simulink library "ddm"  (R2021b)
settings: Solver=VariableStepAuto  StartTime=0.0  StopTime=10.0  RelTol=1e-3
undefined symbols (not defined in the file or in its folder): ADDM_FrTMTqDev_X_Nm, ADDM_RrTMTqDev_X_Nm, ENUM_ADASACCSTA_ERROR, ENUM_ADASACCSTA_OFF, ENUM_ADASACCSTA_STANDBY, ENUM_ALLOWMOV_ALLOWREADY, ENUM_APS, ENUM_BRKSTA_ERROR, ENUM_BRKSTA_OFF, ENUM_BRKSTA_ON, ENUM_BRKSW_INVALID, ENUM_BRKSW_OFF, ENUM_BRKSW_ON, ENUM_CHGPREACTERRSTA_OBCPRE, ENUM_DCDCFAULTSTA_ANYFAULTLV1, ENUM_DCDCFAULTSTA_ANYFAULTLV2, ENUM_DRIVETRAIN_AWD, ENUM_DRIVETRAIN_FWD, ENUM_DRIVETRAIN_RWD, ENUM_EDUDRTSTA_NORMAL, ENUM_EPBSTA_APPLIED, ENUM_EPBSTA_RELEASED, ENUM_ESCAPSSta_APSUNAVAILABLE, ENUM_GEARACTUALPOSN_INVALID, ENUM_GEARACTUALPOSN_P, ENUM_HVBATTREADYPRE_READY, ENUM_MCUWARN_LV0, ENUM_MCUWARN_LV1, ENUM_MCUWARN_LV2, ENUM_MCUWARN_LV3, ENUM_MCUWARN_NOERROR, ENUM_OBCFAULTSTA_ANYFAULT, ENUM_PAS_R2F2, ENUM_PDFAULT_BATTPDFAIL, ENUM_PDFAULT_DCDCDISABLE, ENUM_PDFAULT_MCUDISABLE, ENUM_PDFAULT_MCUDISCHRG, ENUM_POWERSTA_OFF, ENUM_POWERSTA_ON, ENUM_POWERSTA_READY, ENUM_POWERSTA_STANDBY, ENUM_PRESSINDI_LOW, ENUM_PUFAULT_BATTUPFAIL, ENUM_PUFAULT_DCDCENABLEFAIL, ENUM_PUFAULT_PRECHRGCHKFAIL, ENUM_PUFAULT_SAFETYCHKFAIL, ENUM_PUSTATE_COMPLETED, ENUM_PWRSTASW_OFF, ENUM_PWRSTASW_OFFA, ENUM_PWRSTASW_OFFCHVCHRG, ENUM_PWRSTASW_OFFCLVCHRG, ENUM_PWRSTASW_ON, ENUM_PWRSTASW_ONHVCHRG, ENUM_PWRSTASW_READY, ENUM_PWRSTASW_STANDBY, ENUM_RAPSErrWarnSta_NORMAL, ENUM_RAPSErrWarnSta_RAPSERRLV1, ENUM_SHIFTCOMMAND_P, ENUM_SHIFTERERRSTA_PBUTTONFAILURE, ENUM_VEHMALFUNLV_2ND ... (+463)
libraries: hcu_lib x529, $bdroot x5, simulink x4
(part 24 of 25)

== system ddm/DDM/DDM/VMC_DDM/FCM1/FCM1 Checksum Error  ==
  note: Test Detection Criteria
  note: Test Pass Criteria
  note: Release Condiction After Decision
  note: Diagnostics and Fault Handling
  task_time_s : Inport
  VDDM_FCM1CSErr_flg : Inport  Port=2
  No_CAN6_BUS_OFF : Inport  Port=3
  VDDM_FCM1NoComCFS_flg : Inport  Port=4
  VPMM_PowerSta_enum : Inport  Port=5
  DTC_clear_request : Inport  Port=6
  Constant : Constant  Value=ENUM_POWERSTA_OFF
  Constant1 : Constant  Value=FALSE
  Constant16 : Constant  Value=ZERO_INT
  Constant2 : Constant  Value=FALSE
  Constant3 : Constant  Value=KDDM_FCM1CSErrDTC_cnt
  Constant40 : Constant  Value=KDDM_FCM1CSErrDTC_cnt
  Constant41 : Constant  Value=KDDM_FCM1CSErrDetTO_s
  Constant49 : Constant  Value=ENUM_POWERSTA_OFF
  Constant5 : Constant  Value=ENUM_POWERSTA_OFF
  Constant52 : Constant  Value=ENUM_POWERSTA_STANDBY
  Constant6 : Constant  Value=KDDM_FCM1CSErrPassTO_s
  Constant7 : Constant  Value=TRUE
  Constant8 : Constant  Value=KDDM_VMCDiagnosisOffSW_flg
  Constant9 : Constant  Value=KDDM_FCM1CSErrPassTO_s
  DTC_Couter2 : hcu_lib/Basic_Blocks/DTC_Couter
  DTC_Info : hcu_lib/Basic_Blocks/DTC_Info
  Equal : RelationalOperator  Operator=~=  OutDataTypeStr=boolean  RndMeth=Simplest
  Equal1 : RelationalOperator  Operator===  OutDataTypeStr=boolean  RndMeth=Simplest
  Equal2 : RelationalOperator  Operator=~=  OutDataTypeStr=boolean  RndMeth=Simplest
  Equal3 : RelationalOperator  OutDataTypeStr=boolean  RndMeth=Simplest
  Equal8 : RelationalOperator  Operator===  OutDataTypeStr=boolean  RndMeth=Simplest
  Logical Operator1 : Logic  Operator=NOT  AllPortsSameDT=off  OutDataTypeStr=boolean
  Logical Operator10 : Logic  Operator=OR  Inputs=4  AllPortsSameDT=off  OutDataTypeStr=boolean
  Logical Operator11 : Logic  AllPortsSameDT=off  OutDataTypeStr=boolean
  Logical Operator16 : Logic  Operator=NOT  AllPortsSameDT=off  OutDataTypeStr=boolean
  Logical Operator2 : Logic  Inputs=3  AllPortsSameDT=off  OutDataTypeStr=boolean
  Logical Operator4 : Logic  Inputs=3  AllPortsSameDT=off  OutDataTypeStr=boolean
  Logical Operator6 : Logic  Operator=NOT  AllPortsSameDT=off  OutDataTypeStr=boolean
  Relational Operator : RelationalOperator  Operator=>  OutDataTypeStr=boolean  RndMeth=Simplest
  Switch2 : Switch  Criteria=u2 ~= 0
  Switch3 : Switch  Criteria=u2 ~= 0
  Switch5 : Switch  Criteria=u2 ~= 0
  Terminator1 : Terminator
  Test Detection Criteria : hcu_lib/Basic_Blocks/Test Detection Criteria
  Timer1 : hcu_lib/Basic_Blocks/Timer
  Unit Delay3 : UnitDelay  SampleTime=-1  HasFrameUpgradeWarning=on
  VDDM_FCM1CSErrCFS_flg : Outport
  VDDM_FCM1CSErrDTC_raw32 : Outport  Port=2
  wires:
  Relational Operator/1 -> Terminator1/1  "VDDM_FCM1CSErrDFS_flg"
  DTC_Couter2/1 -> [VDDM_FCM1CSErrCFS_flg]  "VDDM_FCM1CSErrCFS_flg"
  [VPMM_PowerSta_enum] -> Unit Delay3/1
  Logical Operator10/1 -> [VDDM_FCM1CSErrCFSRls_flg]  "VDDM_FCM1CSErrCFSRls_flg"
  [VPMM_PowerSta_enum] -> Equal8/1
  [DTC_clear_request] -> Logical Operator10/2
  [VDDM_FCM1CSErrPass_flg] -> Logical Operator10/3
  Constant8/1 -> Logical Operator10/4
  Equal1/1 -> Logical Operator11/1
  Logical Operator11/1 -> Logical Operator10/1
  Unit Delay3/1 -> Equal1/1
  Constant52/1 -> Equal8/2
  DTC_Couter2/2 -> Relational Operator/1  "VDDM_FCM1CSErrDTC_cnt"
  Equal8/1 -> Logical Operator11/2
  Constant49/1 -> Equal1/2
  Constant16/1 -> Relational Operator/2
  Constant3/1 -> DTC_Couter2/3
  [VDDM_FCM1CSErrCFSRls_flg] -> DTC_Couter2/2
  [VDDM_FCM1CSErrDet_flg] -> DTC_Couter2/1
  DTC_Info/1 -> VDDM_FCM1CSErrDTC_raw32/1
  [DTC_clear_request] -> DTC_Info/4
  [VDDM_FCM1CSErrCFS_flg] -> DTC_Info/3
  [VDDM_FCM1CSErrPass_flg] -> DTC_Info/2
  [VDDM_FCM1CSErrDet_flg] -> DTC_Info/1
  Switch5/1 -> Test Detection Criteria/1
  [VDDM_FCM1CSErrCFSRls_flg] -> Switch5/2
  Constant1/1 -> Switch5/1
  Switch2/1 -> Switch5/3
  [task_time_s] -> Timer1/3
  VDDM_FCM1NoComCFS_flg/1 -> [VDDM_FCM1NoComCFS_flg]
  [No_CAN6_BUS_OFF] -> Logical Operator2/1
  Logical Operator16/1 -> Logical Operator2/2
  [VDDM_FCM1NoComCFS_flg] -> Logical Operator16/1
  Constant9/1 -> Timer1/4
  task_time_s/1 -> [task_time_s]  "task_time_s"
  Constant40/1 -> Test Detection Criteria/3
  Constant6/1 -> Equal3/2
  Equal3/1 -> [VDDM_FCM1CSErrPass_flg]  "VDDM_FCM1CSErrPass_flg"
  Equal/1 -> Logical Operator2/3
  Equal2/1 -> Logical Operator4/2
  [No_CAN6_BUS_OFF] -> Logical Operator4/1
  [VPMM_PowerSta_enum] -> Equal2/1
  [VDDM_FCM1CSErr_flg] -> Switch3/1
  Constant/1 -> Equal/2
  Switch3/1 -> Timer1/2, Logical Operator6/1
  [VPMM_PowerSta_enum] -> Equal/1
  Constant41/1 -> Test Detection Criteria/4
  [task_time_s] -> Test Detection Criteria/2
  Test Detection Criteria/1 -> [VDDM_FCM1CSErrDet_flg]  "VDDM_FCM1CSErrDet_flg"
  Logical Operator2/1 -> Switch2/2
  Timer1/1 -> Equal3/1
  [VDDM_FCM1CSErr_flg] -> Switch2/1
  Constant7/1 -> Switch3/3
  Logical Operator4/1 -> Switch3/2
  Constant2/1 -> Switch2/3
  Constant5/1 -> Equal2/2
  Logical Operator6/1 -> Timer1/1
  [VDDM_FCM1CSErrCFS_flg] -> VDDM_FCM1CSErrCFS_flg/1
  VDDM_FCM1CSErr_flg/1 -> [VDDM_FCM1CSErr_flg]
  No_CAN6_BUS_OFF/1 -> [No_CAN6_BUS_OFF]
  DTC_clear_request/1 -> [DTC_clear_request]
  VPMM_PowerSta_enum/1 -> [VPMM_PowerSta_enum]
  Logical Operator1/1 -> Logical Operator4/3
  [VDDM_FCM1NoComCFS_flg] -> Logical Operator1/1

== system ddm/DDM/DDM/VMC_DDM/FCM1/FCM1 Lost Com ==
  note: Release Condiction After Decision
  note: Diagnostics and Fault Handling
  note: Test Detection Criteria
  note: Test Pass Criteria
  task_time_s : Inport
  VDDM_FCM1NoCom_flg : Inport  Port=2
  No_CAN6_BUS_OFF : Inport  Port=3
  VPMM_PowerSta_enum : Inport  Port=4
  DTC_clear_request : Inport  Port=5
  Constant : Constant  Value=ENUM_POWERSTA_OFF
  Constant1 : Constant  Value=FALSE
  Constant10 : Constant  Value=KDDM_FCM1NoComDTC_cnt
  Constant2 : Constant  Value=FALSE
  Constant3 : Constant  Value=KDDM_VMCDiagnosisOffSW_flg
  Constant40 : Constant  Value=KDDM_FCM1NoComDTC_cnt
  Constant41 : Constant  Value=KDDM_FCM1NoComDetTO_s
  Constant49 : Constant  Value=ENUM_POWERSTA_OFF
  Constant5 : Constant  Value=ENUM_POWERSTA_OFF
  Constant52 : Constant  Value=ENUM_POWERSTA_STANDBY
  Constant6 : Constant  Value=KDDM_FCM1NoComPassTO_s
  Constant7 : Constant  Value=TRUE
  Constant8 : Constant  Value=ZERO_INT
  Constant9 : Constant  Value=KDDM_FCM1NoComPassTO_s
  DTC_Couter2 : hcu_lib/Basic_Blocks/DTC_Couter
  DTC_Info : hcu_lib/Basic_Blocks/DTC_Info
  Equal : RelationalOperator  Operator=~=  OutDataTypeStr=boolean  RndMeth=Simplest
  Equal1 : RelationalOperator  Operator===  OutDataTypeStr=boolean  RndMeth=Simplest
  Equal2 : RelationalOperator  Operator=~=  OutDataTypeStr=boolean  RndMeth=Simplest
  Equal3 : RelationalOperator  OutDataTypeStr=boolean  RndMeth=Simplest
  Equal8 : RelationalOperator  Operator===  OutDataTypeStr=boolean  RndMeth=Simplest
  Logical Operator10 : Logic  Operator=OR  Inputs=4  AllPortsSameDT=off  OutDataTypeStr=boolean
  Logical Operator11 : Logic  AllPortsSameDT=off  OutDataTypeStr=boolean
  Logical Operator2 : Logic  AllPortsSameDT=off  OutDataTypeStr=boolean
  Logical Operator4 : Logic  AllPortsSameDT=off  OutDataTypeStr=boolean
  Logical Operator6 : Logic  Operator=NOT  AllPortsSameDT=off  OutDataTypeStr=boolean
  Relational Operator : RelationalOperator  Operator=>  OutDataTypeStr=boolean  RndMeth=Simplest
  Switch2 : Switch  Criteria=u2 ~= 0
  Switch3 : Switch  Criteria=u2 ~= 0
  Switch5 : Switch  Criteria=u2 ~= 0
  Terminator : Terminator
  Test Detection Criteria : hcu_lib/Basic_Blocks/Test Detection Criteria
  Timer1 : hcu_lib/Basic_Blocks/Timer
  Unit Delay3 : UnitDelay  SampleTime=-1  HasFrameUpgradeWarning=on
  VDDM_FCM1NoComCFS_flg : Outport
  VDDM_FCM1NoComDTC_raw32 : Outport  Port=2
  wires:
  [VDDM_FCM1NoComPass_flg] -> Logical Operator10/3
  Constant10/1 -> DTC_Couter2/3
  [VDDM_FCM1NoComCFSRls_flg] -> DTC_Couter2/2
  [VDDM_FCM1NoComDet_flg] -> DTC_Couter2/1
  Relational Operator/1 -> Terminator/1  "VDDM_FCM1NoComDFS_flg"
  DTC_Couter2/1 -> [VDDM_FCM1NoComCFS_flg]  "VDDM_FCM1NoComCFS_flg"
  [VPMM_PowerSta_enum] -> Equal8/1
  [DTC_clear_request] -> Logical Operator10/2
  Equal8/1 -> Logical Operator11/2
  [VPMM_PowerSta_enum] -> Unit Delay3/1
  Logical Operator10/1 -> [VDDM_FCM1NoComCFSRls_flg]  "VDDM_FCM1NoComCFSRls_flg"
  Logical Operator11/1 -> Logical Operator10/1
  Constant49/1 -> Equal1/2
  Unit Delay3/1 -> Equal1/1
  Equal1/1 -> Logical Operator11/1
  DTC_Couter2/2 -> Relational Operator/1  "VDDM_FCM1NoComDTC_cnt"
  Constant3/1 -> Logical Operator10/4
  Constant52/1 -> Equal8/2
  Constant8/1 -> Relational Operator/2
  DTC_Info/1 -> VDDM_FCM1NoComDTC_raw32/1
  [DTC_clear_request] -> DTC_Info/4
  [VDDM_FCM1NoComCFS_flg] -> DTC_Info/3
  [VDDM_FCM1NoComPass_flg] -> DTC_Info/2
  [VDDM_FCM1NoComDet_flg] -> DTC_Info/1
  Constant1/1 -> Switch5/1
  [VDDM_FCM1NoComCFSRls_flg] -> Switch5/2
  Switch5/1 -> Test Detection Criteria/1
  [task_time_s] -> Timer1/3
  Constant9/1 -> Timer1/4
  task_time_s/1 -> [task_time_s]  "task_time_s"
  Constant40/1 -> Test Detection Criteria/3
  Constant6/1 -> Equal3/2
  Equal3/1 -> [VDDM_FCM1NoComPass_flg]  "VDDM_FCM1NoComPass_flg"
  Equal/1 -> Logical Operator2/2
  Equal2/1 -> Logical Operator4/2
  [No_CAN6_BUS_OFF] -> Logical Operator4/1
  [VPMM_PowerSta_enum] -> Equal2/1
  [VDDM_FCM1NoCom_flg] -> Switch3/1
  Switch2/1 -> Switch5/3
  Constant/1 -> Equal/2
  Switch3/1 -> Timer1/2, Logical Operator6/1
  [VPMM_PowerSta_enum] -> Equal/1
  Constant41/1 -> Test Detection Criteria/4
  [task_time_s] -> Test Detection Criteria/2
  Test Detection Criteria/1 -> [VDDM_FCM1NoComDet_flg]  "VDDM_FCM1NoComDet_flg"
  Logical Operator2/1 -> Switch2/2
  Timer1/1 -> Equal3/1
  [VDDM_FCM1NoCom_flg] -> Switch2/1
  Constant7/1 -> Switch3/3
  Logical Operator4/1 -> Switch3/2
  Constant2/1 -> Switch2/3
  Constant5/1 -> Equal2/2
  [No_CAN6_BUS_OFF] -> Logical Operator2/1
  Logical Operator6/1 -> Timer1/1
  [VDDM_FCM1NoComCFS_flg] -> VDDM_FCM1NoComCFS_flg/1
  VDDM_FCM1NoCom_flg/1 -> [VDDM_FCM1NoCom_flg]
  No_CAN6_BUS_OFF/1 -> [No_CAN6_BUS_OFF]
  DTC_clear_request/1 -> [DTC_clear_request]
  VPMM_PowerSta_enum/1 -> [VPMM_PowerSta_enum]

== system ddm/DDM/DDM/VMC_DDM/FCM1/FCM1 Rolling Count Error  ==
  note: Test Detection Criteria
  note: Test Pass Criteria
  note: Release Condiction After Decision
  note: Diagnostics and Fault Handling
  task_time_s : Inport
  VDDM_FCM1RCErr_flg : Inport  Port=2
  No_CAN6_BUS_OFF : Inport  Port=3
  VDDM_FCM1NoComCFS_flg : Inport  Port=4
  VPMM_PowerSta_enum : Inport  Port=5
  DTC_clear_request : Inport  Port=6
  Constant : Constant  Value=ENUM_POWERSTA_OFF
  Constant1 : Constant  Value=FALSE
  Constant16 : Constant  Value=ZERO_INT
  Constant2 : Constant  Value=FALSE
  Constant3 : Constant  Value=KDDM_FCM1RCErrDTC_cnt
  Constant40 : Constant  Value=KDDM_FCM1RCErrDTC_cnt
  Constant41 : Constant  Value=KDDM_FCM1RCErrDetTO_s
  Constant49 : Constant  Value=ENUM_POWERSTA_OFF
  Constant5 : Constant  Value=ENUM_POWERSTA_OFF
  Constant52 : Constant  Value=ENUM_POWERSTA_STANDBY
  Constant6 : Constant  Value=KDDM_FCM1RCErrPassTO_s
  Constant7 : Constant  Value=TRUE
  Constant8 : Constant  Value=KDDM_VMCDiagnosisOffSW_flg
  Constant9 : Constant  Value=KDDM_FCM1RCErrPassTO_s
  DTC_Couter2 : hcu_lib/Basic_Blocks/DTC_Couter
  DTC_Info : hcu_lib/Basic_Blocks/DTC_Info
  Equal : RelationalOperator  Operator=~=  OutDataTypeStr=boolean  RndMeth=Simplest
  Equal1 : RelationalOperator  Operator===  OutDataTypeStr=boolean  RndMeth=Simplest
  Equal2 : RelationalOperator  Operator=~=  OutDataTypeStr=boolean  RndMeth=Simplest
  Equal3 : RelationalOperator  OutDataTypeStr=boolean  RndMeth=Simplest
  Equal8 : RelationalOperator  Operator===  OutDataTypeStr=boolean  RndMeth=Simplest
  From6 : From  Commented=on  GotoTag=VDDM_EDriveSysErrVCUErr_flg
  Logical Operator10 : Logic  Operator=OR  Inputs=4  AllPortsSameDT=off  OutDataTypeStr=boolean
  Logical Operator11 : Logic  AllPortsSameDT=off  OutDataTypeStr=boolean
  Logical Operator16 : Logic  Operator=NOT  AllPortsSameDT=off  OutDataTypeStr=boolean
  Logical Operator2 : Logic  Inputs=3  AllPortsSameDT=off  OutDataTypeStr=boolean
  Logical Operator4 : Logic  AllPortsSameDT=off  OutDataTypeStr=boolean
  Logical Operator6 : Logic  Operator=NOT  AllPortsSameDT=off  OutDataTypeStr=boolean
  Relational Operator : RelationalOperator  Operator=>  OutDataTypeStr=boolean  RndMeth=Simplest
  Switch2 : Switch  Criteria=u2 ~= 0
  Switch3 : Switch  Criteria=u2 ~= 0
  Switch5 : Switch  Criteria=u2 ~= 0
  Terminator : Terminator
  Terminator1 : Terminator
  Test Detection Criteria : hcu_lib/Basic_Blocks/Test Detection Criteria
  Timer1 : hcu_lib/Basic_Blocks/Timer
  Unit Delay3 : UnitDelay  SampleTime=-1  HasFrameUpgradeWarning=on
  VDDM_FCM1RCErrCFS_flg : Outport
  VDDM_FCM1RCErrDTC_raw32 : Outport  Port=2
  wires:
  Relational Operator/1 -> Terminator1/1  "VDDM_FCM1RCErrDFS_flg"
  Constant3/1 -> DTC_Couter2/3
  Equal8/1 -> Logical Operator11/2
  Constant16/1 -> Relational Operator/2
  [VDDM_FCM1RCErrPass_flg] -> Logical Operator10/3
  [VDDM_FCM1RCErrCFSRls_flg] -> DTC_Couter2/2
  Logical Operator10/1 -> [VDDM_FCM1RCErrCFSRls_flg]  "VDDM_FCM1RCErrCFSRls_flg"
  [VDDM_FCM1RCErrDet_flg] -> DTC_Couter2/1
  Constant52/1 -> Equal8/2
  DTC_Couter2/2 -> Relational Operator/1  "VDDM_FCM1RCErrDTC_cnt"
  Constant49/1 -> Equal1/2
  Logical Operator11/1 -> Logical Operator10/1
  Unit Delay3/1 -> Equal1/1
  Equal1/1 -> Logical Operator11/1
  Constant8/1 -> Logical Operator10/4
  [VPMM_PowerSta_enum] -> Equal8/1
  [DTC_clear_request] -> Logical Operator10/2
  [VPMM_PowerSta_enum] -> Unit Delay3/1
  DTC_Couter2/1 -> [VDDM_FCM1RCErrCFS_flg]  "VDDM_FCM1RCErrCFS_flg"
  DTC_Info/1 -> VDDM_FCM1RCErrDTC_raw32/1
  [DTC_clear_request] -> DTC_Info/4
  [VDDM_FCM1RCErrCFS_flg] -> DTC_Info/3
  [VDDM_FCM1RCErrPass_flg] -> DTC_Info/2
  [VDDM_FCM1RCErrDet_flg] -> DTC_Info/1
  Switch5/1 -> Test Detection Criteria/1
  Constant1/1 -> Switch5/1
  [VDDM_FCM1RCErrCFSRls_flg] -> Switch5/2
  [task_time_s] -> Timer1/3
  VDDM_FCM1NoComCFS_flg/1 -> [VDDM_FCM1NoComCFS_flg]
  [No_CAN6_BUS_OFF] -> Logical Operator2/1
  Logical Operator16/1 -> Logical Operator2/2
  [VDDM_FCM1NoComCFS_flg] -> Logical Operator16/1
  Constant9/1 -> Timer1/4
  task_time_s/1 -> [task_time_s]  "task_time_s"
  Constant40/1 -> Test Detection Criteria/3
  Constant6/1 -> Equal3/2
  Equal3/1 -> [VDDM_FCM1RCErrPass_flg]  "VDDM_FCM1RCErrPass_flg"
  Equal/1 -> Logical Operator2/3
  Equal2/1 -> Logical Operator4/2
  [No_CAN6_BUS_OFF] -> Logical Operator4/1
  [VPMM_PowerSta_enum] -> Equal2/1
  [VDDM_FCM1RCErr_flg] -> Switch3/1
  Switch2/1 -> Switch5/3
  Constant/1 -> Equal/2
  Switch3/1 -> Timer1/2, Logical Operator6/1
  [VPMM_PowerSta_enum] -> Equal/1
  Constant41/1 -> Test Detection Criteria/4
  [task_time_s] -> Test Detection Criteria/2
  Test Detection Criteria/1 -> [VDDM_FCM1RCErrDet_flg]  "VDDM_FCM1RCErrDet_flg"
  Logical Operator2/1 -> Switch2/2
  Timer1/1 -> Equal3/1
  [VDDM_FCM1RCErr_flg] -> Switch2/1
  Constant7/1 -> Switch3/3
  Logical Operator4/1 -> Switch3/2
  Constant2/1 -> Switch2/3
  Constant5/1 -> Equal2/2
  Logical Operator6/1 -> Timer1/1
  From6/1 -> Terminator/1
  [VDDM_FCM1RCErrCFS_flg] -> VDDM_FCM1RCErrCFS_flg/1
  VDDM_FCM1RCErr_flg/1 -> [VDDM_FCM1RCErr_flg]
  No_CAN6_BUS_OFF/1 -> [No_CAN6_BUS_OFF]
  DTC_clear_request/1 -> [DTC_clear_request]
  VPMM_PowerSta_enum/1 -> [VPMM_PowerSta_enum]

== system ddm/DDM/DDM/VMC_DDM/FCMACC Signal Error/FCMACC Signal Error  ==
  note: Test Detection Criteria
  note: Test Pass Criteria
  note: Diagnostics and Fault Handling
  note: Release Condiction After Decision
  task_time_s : Inport
  VDDM_FCM1NoComCFS_flg : Inport  Port=2
  VDDM_FCM1RCErrCFS_flg : Inport  Port=3
  VDDM_FCM1CSErrCFS_flg : Inport  Port=4
  No_CAN6_BUS_OFF : Inport  Port=5
  VPMM_PowerSta_enum : Inport  Port=6
  VINP_ADASACCSta_enum : Inport  Port=7
  DTC_clear_request : Inport  Port=8
  VTQD_ExternalTqAllow_flg : Inport  Port=9
  VTQD_ExtDoorAllow_flg : Inport  Port=10
  AND : Logic  Inputs=3  AllPortsSameDT=off  OutDataTypeStr=boolean
  Constant : Constant  Value=ENUM_POWERSTA_OFF
  Constant1 : Constant  Value=ENUM_POWERSTA_OFF
  Constant10 : Constant  Value=ZERO_INT
  Constant12 : Constant  Value=KDDM_FCMACCSigErrDTC_cnt
  Constant16 : Constant  Value=ENUM_ADASACCSTA_STANDBY
  Constant18 : Constant  Value=ENUM_POWERSTA_OFF
  Constant{2,5,19,24} (4 alike) : Constant  Value=FALSE
  Constant20 : Constant  Value=ENUM_POWERSTA_STANDBY
  Constant21 : Constant  Value=TRUE
  Constant25 : Constant  Value=KDDM_VMCDiagnosisOffSW_flg
  Constant3 : Constant  Value=ENUM_ADASACCSTA_ERROR
  Constant4 : Constant  Value=KDDM_FCMACCSigErrDetTO_s
  Constant6 : Constant  Value=KDDM_FCMACCSigErrPassTO_s
  Constant7 : Constant  Value=KDDM_FCMACCSigErrDTC_cnt
  Constant8 : Constant  Value=ENUM_ADASACCSTA_OFF
  Constant9 : Constant  Value=KDDM_FCMACCSigErrPassTO_s
  DTC_Couter1 : hcu_lib/Basic_Blocks/DTC_Couter
  DTC_Info : hcu_lib/Basic_Blocks/DTC_Info
  Equal : RelationalOperator  Operator=~=  OutDataTypeStr=boolean  RndMeth=Simplest
  Equal1 : RelationalOperator  Operator=~=  OutDataTypeStr=boolean  RndMeth=Simplest
  Equal{2,4..5,8..9} (5 alike) : RelationalOperator  Operator===  OutDataTypeStr=boolean  RndMeth=Simplest
  Equal3 : RelationalOperator  OutDataTypeStr=boolean  RndMeth=Simplest
  Logical Operator1 : Logic  Operator=OR  Inputs=4  AllPortsSameDT=off  OutDataTypeStr=boolean
  Logical Operator10 : Logic  AllPortsSameDT=off  OutDataTypeStr=boolean
  Logical Operator{3,5,11..12,14,17..18} (7 alike) : Logic  Operator=NOT  AllPortsSameDT=off  OutDataTypeStr=boolean
  Logical Operator13 : Logic  Inputs=5  AllPortsSameDT=off  OutDataTypeStr=boolean
  Logical Operator2 : Logic  Inputs=5  AllPortsSameDT=off  OutDataTypeStr=boolean
  Logical Operator4 : Logic  Operator=OR  AllPortsSameDT=off  OutDataTypeStr=boolean
  Relational Operator : RelationalOperator  Operator=>  OutDataTypeStr=boolean  RndMeth=Simplest
  Switch{2..3,5..6} (4 alike) : Switch  Criteria=u2 ~= 0
  Terminator : Terminator
  Test Detection Criteria : hcu_lib/Basic_Blocks/Test Detection Criteria
  Timer1 : hcu_lib/Basic_Blocks/Timer
  Unit Delay1 : UnitDelay  SampleTime=-1  HasFrameUpgradeWarning=on
  VDDM_FCMACCSigErrCFS_flg : Outport
  VDDM_FCMACCSigErrDetDTC_raw32 : Outport  Port=2
  wires:
  Switch2/1 -> Switch5/3
  Equal3/1 -> [VDDM_FCMACCSigErrPass_flg]  "VDDM_FCMACCSigErrPass_flg"
  [VDDM_FCMACCSigErrCFS_flg] -> VDDM_FCMACCSigErrCFS_flg/1
  Constant6/1 -> Equal3/2
  [No_CAN6_BUS_OFF] -> Logical Operator2/1
  Logical Operator2/1 -> Switch2/2
  Switch3/1 -> Timer1/1, Logical Operator14/1
  Constant2/1 -> Switch2/3
  Timer1/1 -> Equal3/1
  VDDM_FCM1NoComCFS_flg/1 -> [VDDM_FCM1NoComCFS_flg]
  DTC_clear_request/1 -> [DTC_clear_request]
  VDDM_FCM1CSErrCFS_flg/1 -> [VDDM_FCM1CSErrCFS_flg]
  VPMM_PowerSta_enum/1 -> [VPMM_PowerSta_enum]
  No_CAN6_BUS_OFF/1 -> [No_CAN6_BUS_OFF]
  [VDDM_FCM1NoComCFS_flg] -> Logical Operator17/1
  [VDDM_FCM1CSErrCFS_flg] -> Logical Operator18/1
  Logical Operator17/1 -> Logical Operator2/2
  Logical Operator18/1 -> Logical Operator2/4
  Logical Operator13/1 -> Switch3/2
  Constant5/1 -> Switch3/3
  task_time_s/1 -> [task_time_s]  "task_time_s"
  [task_time_s] -> Test Detection Criteria/2
  Constant7/1 -> Test Detection Criteria/3
  Test Detection Criteria/1 -> [VDDM_FCMACCSigErrDet_flg]  "VDDM_FCMACCSigErrDet_flg"
  Constant9/1 -> Timer1/4
  Equal/1 -> Logical Operator2/5
  VINP_ADASACCSta_enum/1 -> [VINP_ADASACCSta_enum]
  [VINP_ADASACCSta_enum] -> Equal5/1
  Constant3/1 -> Equal5/2
  [VINP_ADASACCSta_enum] -> Equal8/1
  Equal8/1 -> Logical Operator4/1
  Constant8/1 -> Equal8/2
  Logical Operator4/1 -> Switch3/1
  Constant16/1 -> Equal9/2
  [VINP_ADASACCSta_enum] -> Equal9/1
  Equal9/1 -> Logical Operator4/2
  [VDDM_FCM1CSErrCFS_flg] -> Logical Operator12/1
  Logical Operator11/1 -> Logical Operator13/2
  [No_CAN6_BUS_OFF] -> Logical Operator13/1
  [VDDM_FCM1NoComCFS_flg] -> Logical Operator11/1
  Equal1/1 -> Logical Operator13/5
  Logical Operator12/1 -> Logical Operator13/4
  Logical Operator14/1 -> Timer1/2
  [VDDM_FCMACCSigErrCFSRls_flg] -> Switch5/2
  Constant19/1 -> Switch5/1
  Switch5/1 -> Test Detection Criteria/1
  [VDDM_FCMACCSigErrDet_flg] -> DTC_Info/1
  [VDDM_FCMACCSigErrPass_flg] -> DTC_Info/2
  [VDDM_FCMACCSigErrCFS_flg] -> DTC_Info/3
  [DTC_clear_request] -> DTC_Info/4
  DTC_Info/1 -> VDDM_FCMACCSigErrDetDTC_raw32/1  "VDDM_FCMACCSigErrDetDTC_raw32"
  VTQD_ExtDoorAllow_flg/1 -> [VTQD_ExtDoorAllow_flg]
  VTQD_ExternalTqAllow_flg/1 -> [VTQD_ExternalTqAllow_flg]
  AND/1 -> Switch2/1
  Equal5/1 -> AND/2
  [VTQD_ExtDoorAllow_flg] -> AND/3
  [VTQD_ExternalTqAllow_flg] -> AND/1
  Constant4/1 -> Test Detection Criteria/4
  [task_time_s] -> Timer1/3
  [VPMM_PowerSta_enum] -> Equal/1
  Constant/1 -> Equal/2
  Constant1/1 -> Equal1/2
  [VPMM_PowerSta_enum] -> Equal1/1
  DTC_Couter1/1 -> [VDDM_FCMACCSigErrCFS_flg]  "VDDM_FCMACCSigErrCFS_flg"
  [VPMM_PowerSta_enum] -> Unit Delay1/1
  Constant24/1 -> Switch6/3
  Equal2/1 -> Logical Operator10/1
  [VDDM_FCMACCSigErrDet_flg] -> DTC_Couter1/1
  Constant12/1 -> DTC_Couter1/3
  Equal4/1 -> Logical Operator10/2
  Relational Operator/1 -> Terminator/1  "VDDM_FCMACCSigErrDFS_flg"
  Constant20/1 -> Equal4/2
  Constant18/1 -> Equal2/2
  DTC_Couter1/2 -> Relational Operator/1  "VDDM_FCMACCSigErrDTC_cnt"
  Switch6/1 -> [VDDM_FCMACCSigErrCFSRls_flg]  "VDDM_FCMACCSigErrCFSRls_flg"
  Logical Operator10/1 -> Logical Operator1/2
  Logical Operator1/1 -> Switch6/2
  Unit Delay1/1 -> Equal2/1
  Constant21/1 -> Switch6/1
  [VDDM_FCMACCSigErrCFSRls_flg] -> DTC_Couter1/2
  [VDDM_FCMACCSigErrPass_flg] -> Logical Operator1/1
  [VPMM_PowerSta_enum] -> Equal4/1
  [DTC_clear_request] -> Logical Operator1/3
  Constant10/1 -> Relational Operator/2
  Constant25/1 -> Logical Operator1/4
  VDDM_FCM1RCErrCFS_flg/1 -> [VDDM_FCM1RCErrCFS_flg]
  Logical Operator3/1 -> Logical Operator2/3
  [VDDM_FCM1RCErrCFS_flg] -> Logical Operator3/1
  [VDDM_FCM1RCErrCFS_flg] -> Logical Operator5/1
  Logical Operator5/1 -> Logical Operator13/3

== system ddm/DDM/DDM/VMC_DDM/MCU_Fr Signal Error/MCU_Fr Signal Error  ==
  note: Diagnostics and Fault Handling
  note: Release Condiction After Decision
  note: Test Pass Criteria
  note: Test Detection Criteria
  task_time_s : Inport
  VDDM_MCUNF1NoComCFS_flg : Inport  Port=2
  VDDM_MCUNF1RCErrCFS_flg : Inport  Port=3
  VDDM_MCUNF1CSErrCFS_flg : Inport  Port=4
  No_CAN3_BUS_OFF : Inport  Port=5
  VPMM_PowerSta_enum : Inport  Port=6
  VINP_MCUWarnFNidec_enum : Inport  Port=7
  DTC_clear_request : Inport  Port=8
  VPMM_DrivetrainSelect_enum : Inport  Port=9
  Constant : Constant  Value=ENUM_POWERSTA_OFF
  Constant1 : Constant  Value=ENUM_POWERSTA_OFF
  Constant10 : Constant  Value=ENUM_MCUWARN_LV3
  Constant12 : Constant  Value=KDDM_FrMCUSigErrDTC_cnt
  Constant16 : Constant  Value=ENUM_MCUWARN_LV3
  Constant17 : Constant  Value=ENUM_MCUWARN_LV0
  Constant18 : Constant  Value=ZERO_INT
  Constant19 : Constant  Value=ENUM_MCUWARN_LV1
  Constant2 : Constant  Value=FALSE
  Constant20 : Constant  Value=FALSE
  Constant24 : Constant  Value=ENUM_MCUWARN_LV0
  Constant25 : Constant  Value=ENUM_MCUWARN_LV2
  Constant26 : Constant  Value=ENUM_DRIVETRAIN_AWD
  Constant27 : Constant  Value=ENUM_DRIVETRAIN_AWD
  Constant28 : Constant  Value=ENUM_DRIVETRAIN_FWD
  Constant29 : Constant  Value=ENUM_DRIVETRAIN_FWD
  Constant3 : Constant  Value=ENUM_MCUWARN_LV1
  Constant30 : Constant  Value=ENUM_POWERSTA_OFF
  Constant31 : Constant  Value=ENUM_POWERSTA_STANDBY
  Constant32 : Constant  Value=TRUE
  Constant37 : Constant  Value=FALSE
  Constant38 : Constant  Value=KDDM_VMCDiagnosisOffSW_flg
  Constant4 : Constant  Value=KDDM_FrMCUSigErrDetTO_s
  Constant5 : Constant  Value=TRUE
  Constant6 : Constant  Value=KDDM_FrMCUSigErrPassTO_s
  Constant7 : Constant  Value=KDDM_FrMCUSigErrDTC_cnt
  Constant8 : Constant  Value=ENUM_MCUWARN_LV2
  Constant9 : Constant  Value=KDDM_FrMCUSigErrPassTO_s
  DTC_Couter1 : hcu_lib/Basic_Blocks/DTC_Couter
  DTC_Info : hcu_lib/Basic_Blocks/DTC_Info
  Equal : RelationalOperator  Operator=~=  OutDataTypeStr=boolean  RndMeth=Simplest
  Equal1 : RelationalOperator  Operator=~=  OutDataTypeStr=boolean  RndMeth=Simplest
  Equal{2,4..5,8..18} (14 alike) : RelationalOperator  Operator===  OutDataTypeStr=boolean  RndMeth=Simplest
  Equal3 : RelationalOperator  OutDataTypeStr=boolean  RndMeth=Simplest
  Logical Operator1 : Logic  Operator=OR  Inputs=4  AllPortsSameDT=off  OutDataTypeStr=boolean
  Logical Operator10 : Logic  AllPortsSameDT=off  OutDataTypeStr=boolean
  Logical Operator16 : Logic  Operator=OR  Inputs=4  AllPortsSameDT=off  OutDataTypeStr=boolean
  Logical Operator{6,17..18,20..22,24} (7 alike) : Logic  Operator=NOT  AllPortsSameDT=off  OutDataTypeStr=boolean
  Logical Operator2 : Logic  Inputs=6  AllPortsSameDT=off  OutDataTypeStr=boolean
  Logical Operator23 : Logic  Inputs=6  AllPortsSameDT=off  OutDataTypeStr=boolean
  Logical Operator4 : Logic  Operator=OR  Inputs=4  AllPortsSameDT=off  OutDataTypeStr=boolean
  OR : Logic  Operator=OR  AllPortsSameDT=off  OutDataTypeStr=boolean
  OR1 : Logic  Operator=OR  AllPortsSameDT=off  OutDataTypeStr=boolean
  Relational Operator : RelationalOperator  Operator=>  OutDataTypeStr=boolean  RndMeth=Simplest
  Switch{2..3,5..6} (4 alike) : Switch  Criteria=u2 ~= 0
  Terminator : Terminator
  Test Detection Criteria : hcu_lib/Basic_Blocks/Test Detection Criteria
  Timer1 : hcu_lib/Basic_Blocks/Timer
  Unit Delay1 : UnitDelay  SampleTime=-1  HasFrameUpgradeWarning=on
  VDDM_FrMCUSigErrCFS_flg : Outport
  VDDM_FrMCUSigErrDetDTC_raw32 : Outport  Port=2
  wires:
  Logical Operator4/1 -> Switch6/2
  Constant18/1 -> Relational Operator/2
  [VDDM_FrMCUSigErrDet_flg] -> DTC_Couter1/1
  Logical Operator10/1 -> Logical Operator4/2
  DTC_Couter1/1 -> [VDDM_FrMCUSigErrCFS_flg]  "VDDM_FrMCUSigErrCFS_flg"
  DTC_Couter1/2 -> Relational Operator/1  "VDDM_FrMCUSigErrDTC_cnt"
  Constant30/1 -> Equal17/2
  [VPMM_PowerSta_enum] -> Equal18/1
  [DTC_clear_request] -> Logical Operator4/3
  Unit Delay1/1 -> Equal17/1
  Relational Operator/1 -> Terminator/1  "VDDM_FrMCUSigErrDFS_flg"
  Constant32/1 -> Switch6/1
  [VDDM_FrMCUSigErrCFSRls_flg] -> DTC_Couter1/2
  [VPMM_PowerSta_enum] -> Unit Delay1/1
  Equal18/1 -> Logical Operator10/2
  Constant31/1 -> Equal18/2
  Constant37/1 -> Switch6/3
  Equal17/1 -> Logical Operator10/1
  Constant12/1 -> DTC_Couter1/3
  Constant38/1 -> Logical Operator4/4
  Switch6/1 -> [VDDM_FrMCUSigErrCFSRls_flg]  "VDDM_FrMCUSigErrCFSRls_flg"
  [VDDM_FrMCUSigErrPass_flg] -> Logical Operator4/1
  Constant29/1 -> Equal16/2
  OR1/1 -> Logical Operator23/1
  Equal14/1 -> OR1/1
  [VPMM_DrivetrainSelect_enum] -> Equal14/1
  Equal16/1 -> OR1/2
  Constant27/1 -> Equal14/2
  [VPMM_DrivetrainSelect_enum] -> Equal16/1
  [No_CAN3_BUS_OFF] -> Logical Operator23/2
  Logical Operator21/1 -> Logical Operator23/3
  Logical Operator22/1 -> Logical Operator23/4
  Logical Operator24/1 -> Logical Operator23/5
  Equal1/1 -> Logical Operator23/6
  OR/1 -> Logical Operator2/1
  Equal13/1 -> OR/1
  Equal15/1 -> OR/2
  [VPMM_DrivetrainSelect_enum] -> Equal15/1
  Constant28/1 -> Equal15/2
  [No_CAN3_BUS_OFF] -> Logical Operator2/2
  Logical Operator17/1 -> Logical Operator2/3
  Logical Operator18/1 -> Logical Operator2/4
  Logical Operator20/1 -> Logical Operator2/5
  Equal/1 -> Logical Operator2/6
  Constant26/1 -> Equal13/2
  [VPMM_DrivetrainSelect_enum] -> Equal13/1
  VPMM_DrivetrainSelect_enum/1 -> [VPMM_DrivetrainSelect_enum]
  Constant25/1 -> Equal10/2
  Equal12/1 -> Logical Operator1/3
  Equal9/1 -> Logical Operator1/1
  Constant16/1 -> Equal12/2
  [VINP_MCUWarnFNidec_enum] -> Equal10/1
  [VINP_MCUWarnFNidec_enum] -> Equal9/1
  Equal10/1 -> Logical Operator1/2
  Constant17/1 -> Equal8/2
  [VINP_MCUWarnFNidec_enum] -> Equal8/1
  Equal8/1 -> Logical Operator1/4
  [VINP_MCUWarnFNidec_enum] -> Equal12/1
  Constant19/1 -> Equal9/2
  Equal11/1 -> Logical Operator16/4
  [VINP_MCUWarnFNidec_enum] -> Equal11/1
  Constant24/1 -> Equal11/2
  DTC_Info/1 -> VDDM_FrMCUSigErrDetDTC_raw32/1  "VDDM_FrMCUSigErrDetDTC_raw32"
  [DTC_clear_request] -> DTC_Info/4
  [VDDM_FrMCUSigErrCFS_flg] -> DTC_Info/3
  [VDDM_FrMCUSigErrPass_flg] -> DTC_Info/2
  [VDDM_FrMCUSigErrDet_flg] -> DTC_Info/1
  Switch5/1 -> Test Detection Criteria/1
  Constant20/1 -> Switch5/1
  [VDDM_FrMCUSigErrCFSRls_flg] -> Switch5/2
  Logical Operator1/1 -> Switch3/1
  Equal5/1 -> Logical Operator16/3
  Equal4/1 -> Logical Operator16/2
  Equal2/1 -> Logical Operator16/1
  Constant10/1 -> Equal5/2
  [VINP_MCUWarnFNidec_enum] -> Equal5/1
  [VINP_MCUWarnFNidec_enum] -> Equal4/1
  Constant8/1 -> Equal4/2
  Constant3/1 -> Equal2/2
  Constant9/1 -> Timer1/4
  [task_time_s] -> Timer1/3
  Test Detection Criteria/1 -> [VDDM_FrMCUSigErrDet_flg]  "VDDM_FrMCUSigErrDet_flg"
  Constant7/1 -> Test Detection Criteria/3
  Constant4/1 -> Test Detection Criteria/4
  [task_time_s] -> Test Detection Criteria/2
  task_time_s/1 -> [task_time_s]  "task_time_s"
  Switch3/1 -> Logical Operator6/1, Timer1/2
  Constant1/1 -> Equal1/2
  [VDDM_MCUNF1CSErrCFS_flg] -> Logical Operator24/1
  [VDDM_MCUNF1RCErrCFS_flg] -> Logical Operator22/1
  Constant5/1 -> Switch3/3
  Logical Operator23/1 -> Switch3/2
  [VPMM_PowerSta_enum] -> Equal1/1
  [VDDM_MCUNF1NoComCFS_flg] -> Logical Operator21/1
  [VINP_MCUWarnFNidec_enum] -> Equal2/1
  Logical Operator16/1 -> Switch2/1
  [VDDM_MCUNF1CSErrCFS_flg] -> Logical Operator20/1
  [VDDM_MCUNF1RCErrCFS_flg] -> Logical Operator18/1
  [VDDM_MCUNF1NoComCFS_flg] -> Logical Operator17/1
  VINP_MCUWarnFNidec_enum/1 -> [VINP_MCUWarnFNidec_enum]
  No_CAN3_BUS_OFF/1 -> [No_CAN3_BUS_OFF]
  VDDM_MCUNF1CSErrCFS_flg/1 -> [VDDM_MCUNF1CSErrCFS_flg]
  VPMM_PowerSta_enum/1 -> [VPMM_PowerSta_enum]
  VDDM_MCUNF1RCErrCFS_flg/1 -> [VDDM_MCUNF1RCErrCFS_flg]
  DTC_clear_request/1 -> [DTC_clear_request]
  VDDM_MCUNF1NoComCFS_flg/1 -> [VDDM_MCUNF1NoComCFS_flg]
  Timer1/1 -> Equal3/1
  [VPMM_PowerSta_enum] -> Equal/1
  Constant2/1 -> Switch2/3
  Constant/1 -> Equal/2
  Logical Operator6/1 -> Timer1/1
  Logical Operator2/1 -> Switch2/2
  Constant6/1 -> Equal3/2
  [VDDM_FrMCUSigErrCFS_flg] -> VDDM_FrMCUSigErrCFS_flg/1
  Equal3/1 -> [VDDM_FrMCUSigErrPass_flg]  "VDDM_FrMCUSigErrPass_flg"
  Switch2/1 -> Switch5/3

== system ddm/DDM/DDM/VMC_DDM/MCU_Rr Signal Error/MCU_Rr Signal Error  ==
  note: Diagnostics and Fault Handling
  note: Release Condiction After Decision
  note: Test Pass Criteria
  note: Test Detection Criteria
  task_time_s : Inport
  VDDM_MCUNR1NoComCFS_flg : Inport  Port=2
  VDDM_MCUNR1RCErrCFS_flg : Inport  Port=3
  VDDM_MCUNR1CSErrCFS_flg : Inport  Port=4
  No_CAN3_BUS_OFF : Inport  Port=5
  VPMM_PowerSta_enum : Inport  Port=6
  VINP_MCUWarnRNidec_enum : Inport  Port=7
  DTC_clear_request : Inport  Port=8
  VPMM_DrivetrainSelect_enum : Inport  Port=9
  Constant : Constant  Value=ENUM_POWERSTA_OFF
  Constant1 : Constant  Value=ENUM_POWERSTA_OFF
  Constant10 : Constant  Value=ENUM_MCUWARN_LV3
  Constant12 : Constant  Value=KDDM_RrMCUSigErrDTC_cnt
  Constant16 : Constant  Value=ENUM_MCUWARN_LV3
  Constant17 : Constant  Value=ENUM_MCUWARN_LV1
  Constant19 : Constant  Value=ENUM_MCUWARN_LV2
  Constant2 : Constant  Value=FALSE
  Constant20 : Constant  Value=FALSE
  Constant21 : Constant  Value=ZERO_INT
  Constant24 : Constant  Value=ENUM_MCUWARN_LV0
  Constant25 : Constant  Value=ENUM_DRIVETRAIN_AWD
  Constant26 : Constant  Value=ENUM_DRIVETRAIN_AWD
  Constant27 : Constant  Value=ENUM_DRIVETRAIN_RWD
  Constant28 : Constant  Value=ENUM_DRIVETRAIN_RWD
  Constant29 : Constant  Value=ENUM_MCUWARN_LV0
  Constant3 : Constant  Value=ENUM_MCUWARN_LV1
  Constant30 : Constant  Value=ENUM_POWERSTA_OFF
  Constant31 : Constant  Value=ENUM_POWERSTA_STANDBY
  Constant32 : Constant  Value=TRUE
  Constant37 : Constant  Value=FALSE
  Constant38 : Constant  Value=KDDM_VMCDiagnosisOffSW_flg
  Constant4 : Constant  Value=KDDM_RrMCUSigErrDetTO_s
  Constant5 : Constant  Value=TRUE
  Constant6 : Constant  Value=KDDM_RrMCUSigErrPassTO_s
  Constant7 : Constant  Value=KDDM_RrMCUSigErrDTC_cnt
  Constant8 : Constant  Value=ENUM_MCUWARN_LV2
  Constant9 : Constant  Value=KDDM_RrMCUSigErrPassTO_s
  DTC_Couter1 : hcu_lib/Basic_Blocks/DTC_Couter
  DTC_Info : hcu_lib/Basic_Blocks/DTC_Info
  Equal : RelationalOperator  Operator=~=  OutDataTypeStr=boolean  RndMeth=Simplest
  Equal1 : RelationalOperator  Operator=~=  OutDataTypeStr=boolean  RndMeth=Simplest
  Equal{2,4..5,8..18} (14 alike) : RelationalOperator  Operator===  OutDataTypeStr=boolean  RndMeth=Simplest
  Equal3 : RelationalOperator  OutDataTypeStr=boolean  RndMeth=Simplest
  Logical Operator1 : Logic  Operator=OR  Inputs=4  AllPortsSameDT=off  OutDataTypeStr=boolean
  Logical Operator10 : Logic  AllPortsSameDT=off  OutDataTypeStr=boolean
  Logical Operator16 : Logic  Operator=OR  Inputs=4  AllPortsSameDT=off  OutDataTypeStr=boolean
  Logical Operator{6,17..18,20..22,24} (7 alike) : Logic  Operator=NOT  AllPortsSameDT=off  OutDataTypeStr=boolean
  Logical Operator2 : Logic  Inputs=6  AllPortsSameDT=off  OutDataTypeStr=boolean
  Logical Operator23 : Logic  Inputs=6  AllPortsSameDT=off  OutDataTypeStr=boolean
  Logical Operator4 : Logic  Operator=OR  Inputs=4  AllPortsSameDT=off  OutDataTypeStr=boolean
  OR : Logic  Operator=OR  AllPortsSameDT=off  OutDataTypeStr=boolean
  OR1 : Logic  Operator=OR  AllPortsSameDT=off  OutDataTypeStr=boolean
  Relational Operator : RelationalOperator  Operator=>  OutDataTypeStr=boolean  RndMeth=Simplest
  Switch{2..3,5..6} (4 alike) : Switch  Criteria=u2 ~= 0
  Terminator : Terminator
  Test Detection Criteria : hcu_lib/Basic_Blocks/Test Detection Criteria
  Timer1 : hcu_lib/Basic_Blocks/Timer
  Unit Delay1 : UnitDelay  SampleTime=-1  HasFrameUpgradeWarning=on
  VDDM_RrMCUSigErrCFS_flg : Outport
  VDDM_RrMCUSigErrDetDTC_raw32 : Outport  Port=2
  wires:
  Logical Operator1/1 -> Switch3/1
  Equal10/1 -> Logical Operator1/3
  Equal16/1 -> Logical Operator1/4
  [VDDM_RrMCUSigErrDet_flg] -> DTC_Couter1/1
  [VPMM_PowerSta_enum] -> Equal18/1
  Logical Operator4/1 -> Switch6/2
  Constant12/1 -> DTC_Couter1/3
  Constant21/1 -> Relational Operator/2
  Equal17/1 -> Logical Operator10/1
  Constant37/1 -> Switch6/3
  Constant38/1 -> Logical Operator4/4
  Constant31/1 -> Equal18/2
  Equal18/1 -> Logical Operator10/2
  [VPMM_PowerSta_enum] -> Unit Delay1/1
  Constant32/1 -> Switch6/1
  Constant30/1 -> Equal17/2
  Unit Delay1/1 -> Equal17/1
  DTC_Couter1/2 -> Relational Operator/1  "VDDM_RrMCUSigErrDTC_cnt"
  Logical Operator10/1 -> Logical Operator4/2
  [DTC_clear_request] -> Logical Operator4/3
  [VDDM_RrMCUSigErrCFSRls_flg] -> DTC_Couter1/2
  DTC_Couter1/1 -> [VDDM_RrMCUSigErrCFS_flg]  "VDDM_RrMCUSigErrCFS_flg"
  Relational Operator/1 -> Terminator/1  "VDDM_RrMCUSigErrDFS_flg"
  Switch6/1 -> [VDDM_RrMCUSigErrCFSRls_flg]  "VDDM_RrMCUSigErrCFSRls_flg"
  [VDDM_RrMCUSigErrPass_flg] -> Logical Operator4/1
  Constant29/1 -> Equal16/2
  [VINP_MCUWarnRNidec_enum] -> Equal16/1
  OR1/1 -> Logical Operator23/1
  [No_CAN3_BUS_OFF] -> Logical Operator23/2
  Logical Operator21/1 -> Logical Operator23/3
  Logical Operator22/1 -> Logical Operator23/4
  Logical Operator24/1 -> Logical Operator23/5
  Equal1/1 -> Logical Operator23/6
  Equal12/1 -> OR1/1
  [VPMM_DrivetrainSelect_enum] -> Equal12/1
  Equal14/1 -> OR1/2
  Constant25/1 -> Equal12/2
  [VPMM_DrivetrainSelect_enum] -> Equal14/1
  Constant27/1 -> Equal14/2
  OR/1 -> Logical Operator2/1
  Equal13/1 -> OR/1
  [VPMM_DrivetrainSelect_enum] -> Equal13/1
  Equal15/1 -> OR/2
  Constant26/1 -> Equal13/2
  [VPMM_DrivetrainSelect_enum] -> Equal15/1
  Constant28/1 -> Equal15/2
  [No_CAN3_BUS_OFF] -> Logical Operator2/2
  Equal/1 -> Logical Operator2/6
  Logical Operator20/1 -> Logical Operator2/5
  Logical Operator18/1 -> Logical Operator2/4
  Logical Operator17/1 -> Logical Operator2/3
  Equal11/1 -> Logical Operator16/4
  [VINP_MCUWarnRNidec_enum] -> Equal11/1
  Constant24/1 -> Equal11/2
  VPMM_DrivetrainSelect_enum/1 -> [VPMM_DrivetrainSelect_enum]
  DTC_Info/1 -> VDDM_RrMCUSigErrDetDTC_raw32/1  "VDDM_RrMCUSigErrDetDTC_raw32"
  [DTC_clear_request] -> DTC_Info/4
  [VDDM_RrMCUSigErrCFS_flg] -> DTC_Info/3
  [VDDM_RrMCUSigErrPass_flg] -> DTC_Info/2
  [VDDM_RrMCUSigErrDet_flg] -> DTC_Info/1
  Switch5/1 -> Test Detection Criteria/1
  Constant20/1 -> Switch5/1
  [VDDM_RrMCUSigErrCFSRls_flg] -> Switch5/2
  [VINP_MCUWarnRNidec_enum] -> Equal10/1
  Constant16/1 -> Equal10/2
  [VINP_MCUWarnRNidec_enum] -> Equal8/1
  Constant17/1 -> Equal8/2
  Equal8/1 -> Logical Operator1/1
  Equal9/1 -> Logical Operator1/2
  Constant19/1 -> Equal9/2
  [VINP_MCUWarnRNidec_enum] -> Equal9/1
  Equal5/1 -> Logical Operator16/3
  Equal4/1 -> Logical Operator16/2
  Equal2/1 -> Logical Operator16/1
  Constant10/1 -> Equal5/2
  [VINP_MCUWarnRNidec_enum] -> Equal5/1
  [VINP_MCUWarnRNidec_enum] -> Equal4/1
  Constant8/1 -> Equal4/2
  Constant3/1 -> Equal2/2
  Constant9/1 -> Timer1/4
  [task_time_s] -> Timer1/3
  Test Detection Criteria/1 -> [VDDM_RrMCUSigErrDet_flg]  "VDDM_RrMCUSigErrDet_flg"
  Constant7/1 -> Test Detection Criteria/3
  Constant4/1 -> Test Detection Criteria/4
  [task_time_s] -> Test Detection Criteria/2
  task_time_s/1 -> [task_time_s]  "task_time_s"
  Switch3/1 -> Logical Operator6/1, Timer1/2
  Constant1/1 -> Equal1/2
  [VDDM_MCUNR1CSErrCFS_flg] -> Logical Operator24/1
  [VDDM_MCUNR1RCErrCFS_flg] -> Logical Operator22/1
  Constant5/1 -> Switch3/3
  Logical Operator23/1 -> Switch3/2
  [VPMM_PowerSta_enum] -> Equal1/1
  [VDDM_MCUNR1NoComCFS_flg] -> Logical Operator21/1
  [VINP_MCUWarnRNidec_enum] -> Equal2/1
  Logical Operator16/1 -> Switch2/1
  [VDDM_MCUNR1CSErrCFS_flg] -> Logical Operator20/1
  [VDDM_MCUNR1RCErrCFS_flg] -> Logical Operator18/1
  [VDDM_MCUNR1NoComCFS_flg] -> Logical Operator17/1
  VINP_MCUWarnRNidec_enum/1 -> [VINP_MCUWarnRNidec_enum]
  No_CAN3_BUS_OFF/1 -> [No_CAN3_BUS_OFF]
  VDDM_MCUNR1CSErrCFS_flg/1 -> [VDDM_MCUNR1CSErrCFS_flg]
  VPMM_PowerSta_enum/1 -> [VPMM_PowerSta_enum]
  VDDM_MCUNR1RCErrCFS_flg/1 -> [VDDM_MCUNR1RCErrCFS_flg]
  DTC_clear_request/1 -> [DTC_clear_request]
  VDDM_MCUNR1NoComCFS_flg/1 -> [VDDM_MCUNR1NoComCFS_flg]
  Timer1/1 -> Equal3/1
  [VPMM_PowerSta_enum] -> Equal/1
  Constant2/1 -> Switch2/3
  Constant/1 -> Equal/2
  Logical Operator6/1 -> Timer1/1
  Logical Operator2/1 -> Switch2/2
  Constant6/1 -> Equal3/2
  [VDDM_RrMCUSigErrCFS_flg] -> VDDM_RrMCUSigErrCFS_flg/1
  Equal3/1 -> [VDDM_RrMCUSigErrPass_flg]  "VDDM_RrMCUSigErrPass_flg"
  Switch2/1 -> Switch5/3

== system ddm/DDM/DDM/VMC_DDM/Shifter Signal Error/Shifter Signal Error  ==
  note: Diagnostics and Fault Handling
  note: Release Condiction After Decision
  note: Test Pass Criteria
  note: Test Detection Criteria
  task_time_s : Inport
  VDDM_Shifter1NoComCFS_flg : Inport  Port=2
  VDDM_Shifter1RCErrCFS_flg : Inport  Port=3
  VDDM_Shifter1CSErrCFS_flg : Inport  Port=4
  No_CAN3_BUS_OFF : Inport  Port=5
  VPMM_PowerSta_enum : Inport  Port=6
  VINP_ShifterFailsta_enum : Inport  Port=7
  DTC_clear_request : Inport  Port=8
  VTQD_GearActualPosn_enum : Inport  Port=9
  Constant : Constant  Value=ENUM_POWERSTA_OFF
  Constant1 : Constant  Value=ENUM_POWERSTA_OFF
  Constant10 : Constant  Value=ZERO_INT
  Constant11 : Constant  Value=KDDM_VMCDiagnosisOffSW_flg
  Constant12 : Constant  Value=ENUM_POWERSTA_OFF
  Constant13 : Constant  Value=ENUM_POWERSTA_STANDBY
  Constant14 : Constant  Value=TRUE
  Constant15 : Constant  Value=FALSE
  Constant16 : Constant  Value=FALSE
  Constant2 : Constant  Value=FALSE
  Constant3 : Constant  Value=ENUM_SHIFTERERRSTA_PBUTTONFAILURE
  Constant34 : Constant  Value=KDDM_ShifterSigErrDTC_cnt
  Constant4 : Constant  Value=KDDM_ShifterSigErrDetTO_s
  Constant5 : Constant  Value=TRUE
  Constant6 : Constant  Value=KDDM_ShifterSigErrPassTO_s
  Constant7 : Constant  Value=KDDM_ShifterSigErrDTC_cnt
  Constant8 : Constant  Value=ENUM_SHIFTERERRSTA_PBUTTONFAILURE
  Constant9 : Constant  Value=KDDM_ShifterSigErrPassTO_s
  DTC_Couter : hcu_lib/Basic_Blocks/DTC_Couter
  DTC_Info : hcu_lib/Basic_Blocks/DTC_Info
  Equal : RelationalOperator  Operator=~=  OutDataTypeStr=boolean  RndMeth=Simplest
  Equal1 : RelationalOperator  Operator=~=  OutDataTypeStr=boolean  RndMeth=Simplest
  Equal2 : RelationalOperator  OutDataTypeStr=boolean  RndMeth=Simplest
  Equal3 : RelationalOperator  OutDataTypeStr=boolean  RndMeth=Simplest
  Equal4 : RelationalOperator  OutDataTypeStr=boolean  RndMeth=Simplest
  Equal6 : RelationalOperator  Operator===  OutDataTypeStr=boolean  RndMeth=Simplest
  Equal7 : RelationalOperator  Operator===  OutDataTypeStr=boolean  RndMeth=Simplest
  Logical Operator{6,17..18,20..22,24} (7 alike) : Logic  Operator=NOT  AllPortsSameDT=off  OutDataTypeStr=boolean
  Logical Operator2 : Logic  Inputs=5  AllPortsSameDT=off  OutDataTypeStr=boolean
  Logical Operator23 : Logic  Inputs=5  AllPortsSameDT=off  OutDataTypeStr=boolean
  Logical Operator8 : Logic  Operator=OR  Inputs=4  AllPortsSameDT=off  OutDataTypeStr=boolean
  Logical Operator9 : Logic  AllPortsSameDT=off  OutDataTypeStr=boolean
  Relational Operator : RelationalOperator  Operator=>  OutDataTypeStr=boolean  RndMeth=Simplest
  Switch{2..5} (4 alike) : Switch  Criteria=u2 ~= 0
  Terminator : Terminator
  Terminator1 : Terminator
  Test Detection Criteria : hcu_lib/Basic_Blocks/Test Detection Criteria
  Timer1 : hcu_lib/Basic_Blocks/Timer
  Unit Delay2 : UnitDelay  SampleTime=-1  HasFrameUpgradeWarning=on
  VDDM_ShifterSigErrCFS_flg : Outport
  VDDM_ShifterSigErrDetDTC_raw32 : Outport  Port=2
  wires:
  DTC_Info/1 -> [VDDM_ShifterSigErrDetDTC_raw32]  "VDDM_ShifterSigErrDetDTC_raw32"
  Switch5/1 -> Test Detection Criteria/1
  [VDDM_ShifterSigErrCFSRls_flg] -> Switch5/2
  Constant16/1 -> Switch5/1
  [DTC_clear_request] -> DTC_Info/4
  [VDDM_ShifterSigErrCFS_flg] -> DTC_Info/3
  [VDDM_ShifterSigErrPass_flg] -> DTC_Info/2
  [VDDM_ShifterSigErrDet_flg] -> DTC_Info/1
  Equal3/1 -> [VDDM_ShifterSigErrPass_flg]  "VDDM_ShifterSigErrPass_flg"
  VTQD_GearActualPosn_enum/1 -> [VTQD_GearActualPosn_enum]
  Constant11/1 -> Logical Operator8/4
  [VDDM_ShifterSigErrDetDTC_raw32] -> VDDM_ShifterSigErrDetDTC_raw32/1
  Constant10/1 -> Relational Operator/2
  [VINP_ShifterFailsta_enum] -> Equal4/1
  Constant8/1 -> Equal4/2
  Switch2/1 -> Switch5/3
  Equal4/1 -> Switch3/1
  Equal2/1 -> Switch2/1
  Constant3/1 -> Equal2/2
  DTC_Couter/1 -> [VDDM_ShifterSigErrCFS_flg]  "VDDM_ShifterSigErrCFS_flg"
  Relational Operator/1 -> Terminator/1  "VDDM_ShifterSigErrDFS_flg"
  [VDDM_ShifterSigErrDet_flg] -> DTC_Couter/1
  [VDDM_ShifterSigErrCFSRls_flg] -> DTC_Couter/2
  Constant34/1 -> DTC_Couter/3
  DTC_Couter/2 -> Relational Operator/1  "VDDM_ShifterSigErrDTC_cnt"
  Constant9/1 -> Timer1/4
  [task_time_s] -> Timer1/3
  Test Detection Criteria/1 -> [VDDM_ShifterSigErrDet_flg]  "VDDM_ShifterSigErrDet_flg"
  Constant7/1 -> Test Detection Criteria/3
  Constant4/1 -> Test Detection Criteria/4
  [task_time_s] -> Test Detection Criteria/2
  task_time_s/1 -> [task_time_s]  "task_time_s"
  Switch3/1 -> Timer1/2, Logical Operator6/1
  Constant1/1 -> Equal1/2
  [No_CAN3_BUS_OFF] -> Logical Operator23/1
  [VDDM_Shifter1CSErrCFS_flg] -> Logical Operator24/1
  Logical Operator21/1 -> Logical Operator23/2
  Logical Operator24/1 -> Logical Operator23/4
  [VDDM_Shifter1RCErrCFS_flg] -> Logical Operator22/1
  Equal1/1 -> Logical Operator23/5
  Constant5/1 -> Switch3/3
  Logical Operator23/1 -> Switch3/2
  [VPMM_PowerSta_enum] -> Equal1/1
  [VDDM_Shifter1NoComCFS_flg] -> Logical Operator21/1
  Logical Operator22/1 -> Logical Operator23/3
  Logical Operator20/1 -> Logical Operator2/4
  Logical Operator18/1 -> Logical Operator2/3
  Logical Operator17/1 -> Logical Operator2/2
  [VINP_ShifterFailsta_enum] -> Equal2/1
  [VDDM_Shifter1CSErrCFS_flg] -> Logical Operator20/1
  [VDDM_Shifter1RCErrCFS_flg] -> Logical Operator18/1
  [VDDM_Shifter1NoComCFS_flg] -> Logical Operator17/1
  Equal/1 -> Logical Operator2/5
  VINP_ShifterFailsta_enum/1 -> [VINP_ShifterFailsta_enum]
  No_CAN3_BUS_OFF/1 -> [No_CAN3_BUS_OFF]
  VDDM_Shifter1CSErrCFS_flg/1 -> [VDDM_Shifter1CSErrCFS_flg]
  VPMM_PowerSta_enum/1 -> [VPMM_PowerSta_enum]
  VDDM_Shifter1RCErrCFS_flg/1 -> [VDDM_Shifter1RCErrCFS_flg]
  DTC_clear_request/1 -> [DTC_clear_request]
  VDDM_Shifter1NoComCFS_flg/1 -> [VDDM_Shifter1NoComCFS_flg]
  Timer1/1 -> Equal3/1
  [VPMM_PowerSta_enum] -> Equal/1
  Logical Operator8/1 -> Switch4/2
  [VPMM_PowerSta_enum] -> Equal7/1
  Constant14/1 -> Switch4/1
  Constant2/1 -> Switch2/3
  Constant12/1 -> Equal6/2
  Unit Delay2/1 -> Equal6/1
  Constant/1 -> Equal/2
  Constant13/1 -> Equal7/2
  Logical Operator6/1 -> Timer1/1
  Logical Operator2/1 -> Switch2/2
  [DTC_clear_request] -> Logical Operator8/3
  [VDDM_ShifterSigErrPass_flg] -> Logical Operator8/1
  [No_CAN3_BUS_OFF] -> Logical Operator2/1
  Switch4/1 -> [VDDM_ShifterSigErrCFSRls_flg]  "VDDM_ShifterSigErrCFSRls_flg"
  Logical Operator9/1 -> Logical Operator8/2
  [VPMM_PowerSta_enum] -> Unit Delay2/1
  Constant6/1 -> Equal3/2
  Equal7/1 -> Logical Operator9/2
  Equal6/1 -> Logical Operator9/1
  Constant15/1 -> Switch4/3
  [VDDM_ShifterSigErrCFS_flg] -> VDDM_ShifterSigErrCFS_flg/1
  [VTQD_GearActualPosn_enum] -> Terminator1/1
